simulink model "ej_figura6"  (R2015b)
settings: Solver=ode45  StartTime=0.0  StopTime=15  RelTol=1e-3
settings Model: Creator=Felix  LastModifiedBy=Felix

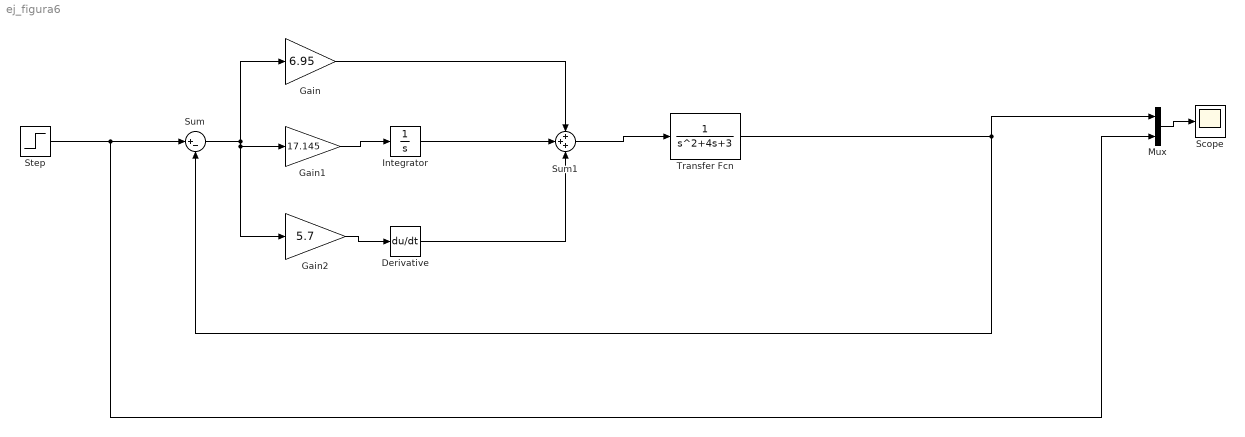
== system ej_figura6 ==
  Derivative : Derivative
  Gain : Gain  Gain=6.95
  Gain1 : Gain  Gain=17.145
  Gain2 : Gain  Gain=5.7
  Integrator : Integrator
  Mux : Mux  Inputs=2
  Scope : Scope
  Step : Step  SampleTime=0
  Sum : Sum  Inputs=|+-
  Sum1 : Sum  Inputs=+++
  Transfer Fcn : TransferFcn  Denominator=[1 4 3]
  wires:
  Sum/1 -> Gain2/1, Gain1/1, Gain/1
  Gain1/1 -> Integrator/1
  Gain2/1 -> Derivative/1
  Gain/1 -> Sum1/1
  Integrator/1 -> Sum1/2
  Derivative/1 -> Sum1/3
  Sum1/1 -> Transfer Fcn/1
  Transfer Fcn/1 -> Mux/1, Sum/2
  Step/1 -> Mux/2, Sum/1
  Mux/1 -> Scope/1
